simulink model "model"  (R2019a)
settings: Solver=FixedStepDiscrete  StartTime=0.0  StopTime=8  FixedStep=1/30  RelTol=1e-3  EnableMultiTasking=on
values from neighbouring files (symbols this model uses):
  A0 = 914.02    [parameter.mat]
  A1 = 12.9    [parameter.mat]
  A2 = 2028.24    [parameter.mat]
  b = 1.14    [parameter.mat]
  bpitch = 4000    [parameter.mat]
  broll = 4000    [parameter.mat]
  c = 1.14    [parameter.mat]
  C1 = 1    [parameter.mat]
  C2 = 0.34    [parameter.mat]
  C3 = 0.57    [parameter.mat]
  C4 = 0.32    [parameter.mat]
  CF = 18.7    [parameter.mat]
  f = 1.215    [parameter.mat]
  Fzt = 810    [parameter.mat]
  hs = 0.55    [parameter.mat]
  ip = 50    [parameter.mat]
  ir = 425    [parameter.mat]
  iw = 1.1    [parameter.mat]
  iz = 3136    [parameter.mat]
  Ka = 0.05    [parameter.mat]
  kpitch = 170000    [parameter.mat]
  kroll = 90000    [parameter.mat]
  m = 750    [parameter.mat]
  miudot = 0.85    [parameter.mat]
  ms = 650    [parameter.mat]
  r = 1.205    [parameter.mat]
  rw = 0.237    [parameter.mat]
  Tp = 24    [parameter.mat]
  Tw = 6    [parameter.mat]
  w = 2.28    [parameter.mat]
undefined symbols (not defined in the file or in its folder): DiscIntNeverNeededParam, Rec, SDTV, sigbuilder_block
libraries: dspmtrx3 x3, visionconversions x2, visiontextngfix x2, visiontransforms x2, fuzblock x1, dspvision x1, visionfilter x1, visionsinks x1, visionstatistics x1
(part 1 of 3)
settings Model: Creator=embb8  LastModifiedBy=embb8
settings SolverCC: PositivePriorityOrder=on
settings DataIOCC: ReturnWorkspaceOutputs=off
settings OptimizationCC: DefaultParameterBehavior=Inlined  LifeSpan=Inf  MaxStackSize=64
settings DebuggingCC: PregeneratedLibrarySubsystemCodeDiagnostic=none  SFUnexpectedBacktrackingDiag=warning  SFNoUnconditionalDefaultTransitionDiag=warning  SFExecutionAtInitializationDiag=none  ArithmeticOperatorsInVariantConditions=warning
settings HardwareCC: UseEmbeddedCoderFeatures=off  UseSimulinkCoderFeatures=off
settings SFSimCC: SimUseLocalCustomCode=off  MATLABDynamicMemAlloc=off
settings RTWCC: SystemTargetFile=ert.tlc  TemplateMakefile=ert_default_tmf  GenerateReport=on  RTWUseLocalCustomCode=off  Toolchain=GNU GCC Raspberry Pi  IncludeHyperlinkInReport=on  LaunchReport=on  GenerateTraceInfo=on  GenerateTraceReport=on  GenerateTraceReportSl=on  GenerateTraceReportSf=on  GenerateTraceReportEml=on
settings CodeAppCC: ForceParamTrailComments=on  IgnoreCustomStorageClasses=off  OperatorAnnotations=on  SimulinkDataObjDesc=on  SFDataObjDesc=on  MATLABFcnDesc=on  InsertBlockDesc=on  StateflowObjectComments=on  MATLABSourceComments=on
settings ERTTargetCC: MultiwordLength=2048  SupportNonInlinedSFcns=on  SupportVariableSizeSignals=on  InlinedParameterPlacement=NonHierarchical  ERTCustomFileTemplate=example_file_process.tlc
settings ConfigComp: CovMetricSettings=dw  CovHtmlReporting=on  CovSaveCumulativeToWorkspaceVar=on  CovSaveSingleToWorkspaceVar=on  CovExternalEMLEnable=off

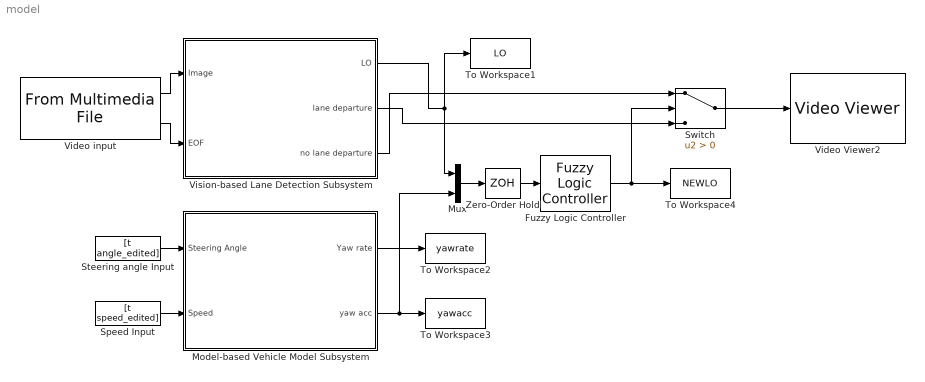
== system model ==
  Fuzzy Logic Controller : fuzblock/Fuzzy Logic  Controller  FIS=ld  OutputSampleNumber=101  DataType=double  FuzzifiedInputs=off  RuleFiringStrengths=off  RuleOutputs=off  AggregatedOutputs=off  SimulateUsing=Interpreted execution  OutOfRangeInputValueMessage=warning  NoRuleFiredMessage=warning  EmptyOutputFuzzySetMessage=warning
  Model-based Vehicle Model Subsystem : Subsystem
  Mux : Mux  Inputs=2
  Speed Input : FromWorkspace  VariableName=[t speed_edited]  SampleTime=0
  Steering angle Input : FromWorkspace  VariableName=[t angle_edited]  SampleTime=0
  Switch : Switch  Criteria=u2 > Threshold
  To Workspace1 : ToWorkspace  VariableName=LO  SampleTime=-1
      settings: Save2DSignal=2-D array (concatenate along first dimension)
  To Workspace2 : ToWorkspace  VariableName=yawrate  SampleTime=-1
      settings: Save2DSignal=2-D array (concatenate along first dimension)
  To Workspace3 : ToWorkspace  VariableName=yawacc  SampleTime=-1
      settings: Save2DSignal=2-D array (concatenate along first dimension)
  To Workspace4 : ToWorkspace  VariableName=NEWLO  SampleTime=-1
      settings: Save2DSignal=2-D array (concatenate along first dimension)
  Video Viewer2 : VideoViewer  FigPos=[617 762 372 213.6]
  Video input : dspvision/From Multimedia File  inputFilename=C:\Users\embb8\Desktop\clip20.avi  readRange=[1 Inf]  loop=on  numPlays=inf  outputStreams=Video only  videoDataType=single  audioDataType=int16  inheritSampleTime=off  userDefinedSampleTime=1/30  noAudioOutput=off  isIntensityVideo=off  fourcc=RGB  colorVideoFormat=One multidimensional signal  outputEOF=on  dataOrg=Column-major  audioFrameSize=1024  computeAudioFrameSize=off  outSamplingMode=Sample based
      settings: SourceProductName=Computer Vision Toolbox  SourceProductBaseCode=VP
  Vision-based Lane Detection Subsystem : Subsystem
  Zero-Order Hold : ZeroOrderHold  SampleTime=1/30
  wires:
  Video input/1 -> Vision-based Lane Detection Subsystem/1(Image)
  Video input/2 -> Vision-based Lane Detection Subsystem/2(EOF)
  Speed Input/1 -> Model-based Vehicle Model Subsystem/2(Speed)
  Steering angle Input/1 -> Model-based Vehicle Model Subsystem/1(Steering Angle)
  Model-based Vehicle Model Subsystem/1(Yaw rate) -> To Workspace2/1
  Vision-based Lane Detection Subsystem/1(LO) -> Mux/1, To Workspace1/1
  Vision-based Lane Detection Subsystem/2(lane departure) -> Switch/3
  Vision-based Lane Detection Subsystem/3(no lane departure) -> Switch/1
  Switch/1 -> Video Viewer2/1
  Model-based Vehicle Model Subsystem/2(yaw acc) -> Mux/2, To Workspace3/1
  Mux/1 -> Zero-Order Hold/1
  Fuzzy Logic Controller/1 -> To Workspace4/1, Switch/2
  Zero-Order Hold/1 -> Fuzzy Logic Controller/1

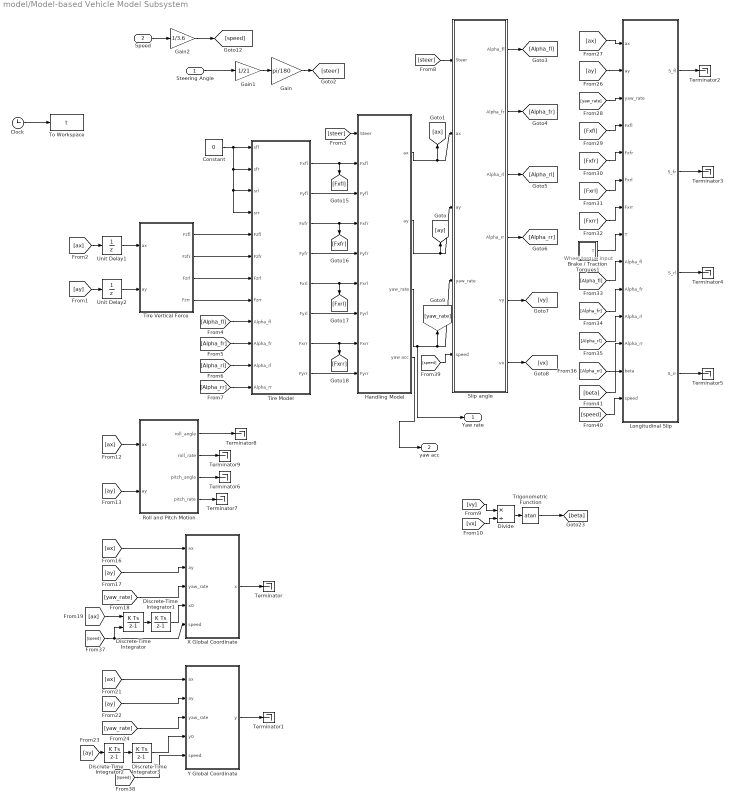
== system model/Model-based Vehicle Model Subsystem ==
  note: Wheel torque input
  Steering Angle : Inport
  Speed : Inport  Port=2
  Brake / Traction Torques1 : Subsystem
  Clock : Clock
  Constant : Constant  Value=0
  Discrete-Time Integrator : DiscreteIntegrator  InitialConditionSource=external  InitialCondition=22.222  SampleTime=-1  LimitOutput=on  LowerSaturationLimit=0  ICPrevOutput=DiscIntNeverNeededParam  ICPrevScaledInput=DiscIntNeverNeededParam
  Discrete-Time Integrator1 : DiscreteIntegrator  SampleTime=-1  LimitOutput=on  LowerSaturationLimit=0  ICPrevOutput=DiscIntNeverNeededParam  ICPrevScaledInput=DiscIntNeverNeededParam
  Discrete-Time Integrator2 : DiscreteIntegrator  SampleTime=-1  ICPrevOutput=DiscIntNeverNeededParam  ICPrevScaledInput=DiscIntNeverNeededParam
  Discrete-Time Integrator3 : DiscreteIntegrator  SampleTime=-1  ICPrevOutput=DiscIntNeverNeededParam  ICPrevScaledInput=DiscIntNeverNeededParam
  Divide : Product  Inputs=*/
  Gain : Gain  Gain=pi/180
  Gain1 : Gain  Gain=1/21
  Gain2 : Gain  Gain=1/3.6
  "Handling Model " : Subsystem
  Longitudinal Slip : Subsystem
  Roll and Pitch Motion : Subsystem
  "Slip angle " : Subsystem
  Terminator{,1..9} (10 alike) : Terminator
  Tire Model : Subsystem
  Tire Vertical Force : Subsystem
  To Workspace : ToWorkspace  VariableName=t  SampleTime=-1
  Trigonometric Function : Trigonometry  Operator=atan
  Unit Delay1 : UnitDelay  SampleTime=1/30  HasFrameUpgradeWarning=on
  Unit Delay2 : UnitDelay  SampleTime=1/30  HasFrameUpgradeWarning=on
  X Global Coordinate : Subsystem
  Y Global Coordinate : Subsystem
  Yaw rate : Outport
  yaw acc : Outport  Port=2
  wires:
  [speed] -> X Global Coordinate/5(speed), Discrete-Time Integrator/2
  [speed] -> Longitudinal Slip/14(speed)
  [Fxrr] -> Longitudinal Slip/7(Fxrr)
  Gain1/1 -> Gain/1
  "Slip angle "/3(Alpha_rl) -> [Alpha_rl]
  Longitudinal Slip/4(S_rr) -> Terminator5/1
  [ax] -> Longitudinal Slip/1(ax)
  Discrete-Time Integrator3/1 -> Y Global Coordinate/4(y0)
  [speed] -> Y Global Coordinate/5(speed)
  [ay] -> X Global Coordinate/2(ay)
  Longitudinal Slip/3(S_rl) -> Terminator4/1
  [Fxfl] -> Longitudinal Slip/4(Fxfl)
  Tire Model/6(Fyrl) -> "Handling Model "/7(Fyrl)
  Y Global Coordinate/1(y) -> Terminator1/1
  [Alpha_rr] -> Longitudinal Slip/12(Alpha_rr)
  Unit Delay2/1 -> Tire Vertical Force/2(ay)
  Tire Vertical Force/2(Fzfr) -> Tire Model/6(Fzfr)
  [Alpha_rr] -> Tire Model/12(Alpha_rr)
  Clock/1 -> To Workspace/1
  Brake / Traction Torques1/1(T) -> Longitudinal Slip/8(T)
  [ax] -> Roll and Pitch Motion/1(ax)
  [ax] -> X Global Coordinate/1(ax)
  Constant/1 -> Tire Model/1(sfl), Tire Model/2(sfr), Tire Model/3(srl), Tire Model/4(srr)
  Roll and Pitch Motion/1(roll_angle) -> Terminator8/1
  [Fxrl] -> Longitudinal Slip/6(Fxrl)
  [ay] -> Longitudinal Slip/2(ay)
  Tire Vertical Force/1(Fzfl) -> Tire Model/5(Fzfl)
  Roll and Pitch Motion/4(pitch_rate) -> Terminator7/1
  [Fxfr] -> Longitudinal Slip/5(Fxfr)
  [yaw_rate] -> Y Global Coordinate/3(yaw_rate)
  [Alpha_fr] -> Longitudinal Slip/10(Alpha_fr)
  Roll and Pitch Motion/3(pitch_angle) -> Terminator6/1
  [Alpha_fl] -> Longitudinal Slip/9(Alpha_fl)
  [Alpha_fl] -> Tire Model/9(Alpha_fl)
  [Alpha_rl] -> Longitudinal Slip/11(Alpha_rl)
  [yaw_rate] -> Longitudinal Slip/3(yaw_rate)
  [yaw_rate] -> X Global Coordinate/3(yaw_rate)
  [beta] -> Longitudinal Slip/13(beta)
  X Global Coordinate/1(x) -> Terminator/1
  [speed] -> "Slip angle "/5(speed)
  [ax] -> Y Global Coordinate/1(ax)
  "Slip angle "/6(vx) -> [vx]
  "Slip angle "/4(Alpha_rr) -> [Alpha_rr]
  [ay] -> Discrete-Time Integrator2/1
  Longitudinal Slip/2(S_fr) -> Terminator3/1
  "Handling Model "/1(ax) -> [ax], "Slip angle "/2(ax)
  Discrete-Time Integrator/1 -> Discrete-Time Integrator1/1
  [steer] -> "Handling Model "/1(Steer)
  "Slip angle "/2(Alpha_fr) -> [Alpha_fr]
  [Alpha_fr] -> Tire Model/10(Alpha_fr)
  [ax] -> Unit Delay1/1
  [ax] -> Discrete-Time Integrator/1
  [ay] -> Roll and Pitch Motion/2(ay)
  Roll and Pitch Motion/2(roll_rate) -> Terminator9/1
  Tire Model/1(Fxfl) -> "Handling Model "/2(Fxfl), [Fxfl]
  Discrete-Time Integrator2/1 -> Discrete-Time Integrator3/1
  Tire Model/8(Fyrr) -> "Handling Model "/9(Fyrr)
  "Handling Model "/2(ay) -> [ay], "Slip angle "/3(ay)
  Gain/1 -> [steer]
  [ay] -> Unit Delay2/1
  [Alpha_rl] -> Tire Model/11(Alpha_rl)
  [ay] -> Y Global Coordinate/2(ay)
  "Slip angle "/1(Alpha_fl) -> [Alpha_fl]
  "Slip angle "/5(vy) -> [vy]
  Tire Model/7(Fxrr) -> "Handling Model "/8(Fxrr), [Fxrr]
  [steer] -> "Slip angle "/1(Steer)
  Tire Vertical Force/4(Fzrr) -> Tire Model/8(Fzrr)
  Longitudinal Slip/1(S_fl) -> Terminator2/1
  Tire Model/2(Fyfl) -> "Handling Model "/3(Fyfl)
  Tire Model/4(Fyfr) -> "Handling Model "/5(Fyfr)
  Discrete-Time Integrator1/1 -> X Global Coordinate/4(x0)
  Tire Model/3(Fxfr) -> "Handling Model "/4(Fxfr), [Fxfr]
  Tire Vertical Force/3(Fzrl) -> Tire Model/7(Fzrl)
  Unit Delay1/1 -> Tire Vertical Force/1(ax)
  Tire Model/5(Fxrl) -> "Handling Model "/6(Fxrl), [Fxrl]
  Speed/1 -> Gain2/1
  Steering Angle/1 -> Gain1/1
  "Handling Model "/3(yaw_rate) -> Yaw rate/1, "Slip angle "/4(yaw_rate), [yaw_rate]
  [vy] -> Divide/1
  [vx] -> Divide/2
  Divide/1 -> Trigonometric Function/1
  Trigonometric Function/1 -> [beta]
  Gain2/1 -> [speed]
  "Handling Model "/4(yaw acc) -> yaw acc/1

== system model/Vision-based Lane Detection Subsystem ==
  note: |
      | |
      | |
      | |
      | |
      | |
      | y(180)
  note: _____________>x(320)
  note: x11 y12 x12 y12
      | x21 y21 x22 y22
  note: Plan to do list:
      | 1. Vision lateral offset (Done)
      | 2. Benchmark with other edge-based lane detection algorithm.
      | 3. Vehicle Model (Driver Model) lateral offset
      | 4. Steering Angle and Speed Sensor integrate into vehicle model.
      | 5. Integrate vision model and vehicle model with fuzzy system to compare respective lateral offset for lane warning.
  Image : Inport
  EOF : Inport  Port=2
  2-D FIR Filter : visionfilter/2-D FIR Filter  separable=off  filtSrc=Specify via dialog  filterMtrx=[-1 0 1]  verticalFilter=[4 0]  horizontalFilter=[4 0]  outSize=Full  padType=Replicate  padSrc=Specify via dialog  padVal=0  method=Convolution  firstCoeffMode=Specify word length  firstCoeffWordLength=16  firstCoeffFracLength=14  firstCoeffSignedness=Signed  firstCoeffLastDataTypeStr=fixdt(1,16)  outputSignedness=Auto  accumLastDataTypeStr=Inherit: Same as product output  prodOutputMode=Binary point scaling  prodOutputWordLength=32  prodOutputFracLength=10  prodOutputLastDataTypeStr=fixdt([],32,10)  roundingMode=Floor  overflowMode=on  firstCoeffDataTypeStr=fixdt(1,16)  firstCoeffMin=[]  firstCoeffMax=[]  prodOutputDataTypeStr=fixdt([],32,10)  accumDataTypeStr=Inherit: Same as product output  outputMin=[]  outputMax=[]
      settings: SourceProductName=Computer Vision Toolbox  SourceProductBaseCode=VP
  After : Display
  Clip image : dspmtrx3/Submatrix  RowSpan=Range of rows  RowStartMode=Index  RowStartIndex=u+1  RowEndMode=Last  RowEndIndex=1  ColSpan=All columns  ColStartMode=First  ColStartIndex=1  ColEndMode=Last  ColEndIndex=1
  Color Space Conversion : visionconversions/Color Space  Conversion  conversion=Obsolete  conversionActive=R'G'B' to intensity  wp_str=D65  rec=Rec. 601 (SDTV)  sys=1125/60/2:1  imagePorts=One multidimensional signal
  Draw Shapes : visiontextngfix/Draw Shapes  shape=Lines  fill=on  lineWidth=3  fillClrSource=Specify via dialog  display=User-specified value  intensity=200  color=[255 0 0]  opacity=0.6  viewport=Entire image  antialiasing=on  inType=Obsolete  imagePorts=One multidimensional signal  roundingMode=Floor  overflowMode=off  memoryMode=Specify word length  memoryWordLength=16  prodOutputMode=Binary point scaling  prodOutputWordLength=32  prodOutputFracLength=14  prodOutputSlope=2^-14  accumSlope=2^-14  memoryFracLength=14
      settings: SourceProductName=Computer Vision Toolbox
  Frame Rate Display : visionsinks/Frame Rate Display  UpdateRate=1
      settings: SourceProductName=Computer Vision Toolbox  SourceProductBaseCode=VP
  Hough Transform : Subsystem
  Image thresholding : visionconversions/Autothreshold  operator=>  threshOut=off  effMetricOut=off  userDefinedRange=off  umin=0  umax=255  outOfRngOpt=Warn and saturate  scaleThreshold=off  scaleFactor=1  roundingMode=Floor  overflowMode=off  P1Mode=Specify word length  P1WordLength=32  P1FracLength=30  P1Slope=2^-30  A1Slope=2^-30  P2Mode=Specify word length  P2WordLength=32  P2FracLength=22  P2Slope=2^-22  A2Slope=2^-22  P3Mode=Specify word length  P3WordLength=32  P3FracLength=14  P3Slope=2^-14  A3Slope=2^-14  P4Mode=Binary point scaling  P4WordLength=32  P4FracLength=15  P4Slope=2^-15  A4Slope=2^-4  Q1Mode=Specify word length  Q1WordLength=32  Q1FracLength=16  Q1Slope=2^-16  EMMode=Specify word length  EMWordLength=16  EMFracLength=14  EMSlope=2^-14
      settings: SourceProductName=Computer Vision Toolbox  SourceProductBaseCode=VP
  Insert Text : visiontextngfix/Insert Text  inputType=Obsolete  theText='Lane Departure'  getTextLocFrom=Specify via dialog  textLoc=[120 60]  getTextColorFrom=Specify via dialog  textColor=[255 0 0]  getTextIntensityFrom=Specify via dialog  textIntensity=0  getTextOpacityFrom=Specify via dialog  textOpacity=1.0  dummyVar2=0  dummyVar3=0  dummyVar4=0  imagePorts=One multidimensional signal  isInputTransposed=off  fontFace=LucidaSansRegular  dummyVar1=0  blockFontSize=20  antiAliased=on
      settings: SourceProductName=Computer Vision Toolbox  SourceProductBaseCode=VP
  Saturation : Saturate  UpperLimit=1  LowerLimit=0
  Selector3 : Selector  NumberOfDimensions=2  InputPortWidth=3  IndexOptions=Select all,Index vector (dialog)  Indices=[2 1],[2 1 4 3]  OutputSizes=1,1
  Selector4 : Selector  NumberOfDimensions=2  InputPortWidth=3  IndexOptions=Index vector (dialog),Select all  Indices=[2 1 4 3],1  OutputSizes=1,1
  Stop Simulation : Stop
  Subsystem : Subsystem
  Transpose : Math  Operator=transpose  SaturateOnIntegerOverflow=on
  Transpose1 : Math  Operator=transpose  SaturateOnIntegerOverflow=on
  coordinate mapping : Subsystem
  lateral offset : Subsystem
  offset (+88) : Subsystem
  LO : Outport
  lane departure : Outport  Port=2
  no lane departure : Outport  Port=3
  wires:
  Subsystem/1(Out1) -> coordinate mapping/1(In1), After/1
  EOF/1 -> Stop Simulation/1
  2-D FIR Filter/1 -> Saturation/1
  Saturation/1 -> Image thresholding/1
  Transpose1/1 -> Subsystem/1(In1), Draw Shapes/2
  Image thresholding/1 -> Hough Transform/1(In1)
  offset (+88)/2(left) -> lateral offset/2(left)
  Hough Transform/1(Out1) -> Selector3/1
  Image/1 -> Draw Shapes/1, Color Space Conversion/1
  offset (+88)/3(right) -> lateral offset/1(right)
  Transpose/1 -> offset (+88)/1(In1)
  offset (+88)/1(Out1) -> Selector4/1
  Clip image/1 -> Hough Transform/2(ref_I), 2-D FIR Filter/1
  Selector4/1 -> Transpose1/1
  Draw Shapes/1 -> no lane departure/1, Insert Text/1, Frame Rate Display/1
  Selector3/1 -> Transpose/1
  Color Space Conversion/1 -> Clip image/1
  Insert Text/1 -> lane departure/1
  lateral offset/1(lateral offset) -> LO/1

== system model/Model-based Vehicle Model Subsystem/Brake // Traction Torques1 ==
  note: T negative for braking
      | T positive for traction
  BRAKE : Subsystem  Tag=STV Subsys  LoadFcn=sigbuilder_block('load');  StartFcn=sigbuilder_block('start');  StopFcn=sigbuilder_block('stop');  ClipboardFcn=sigbuilder_block('clipboard');  mask(Sigbuilder block){tuvar=[0:10]}
      mask help: Sigbuilder GUI
      mask init:
      | if ~strcmp(get_param(bdroot(gcbh),'SimulationStatus'),'stopped') tuvar = sigbuilder_block('maskInit'); end
      settings: CopyFcn=sigbuilder_block('copy');  DeleteFcn=sigbuilder_block('delete');  ModelCloseFcn=sigbuilder_block('modelClose');  PreSaveFcn=sigbuilder_block('preSave');  PauseFcn=sigbuilder_block('pause')  ContinueFcn=sigbuilder_block('continue')  NameChangeFcn=sigbuilder_block('namechange');  OpenFcn=sigbuilder_block('open',[51.75 84.75 550.5 363.75 ]);  CloseFcn=sigbuilder_block('close');
      mask Display: plot(0, 0, 100, 100,[2, 2, 32, 32, 2], [68, 8, 8, 68, 68],[32, 2], [38, 38], [32, 19, 2],[53, 60, 44], [32, 17, 17, 2],[16, 16, 31, 31]);txt = getActiveGroup(gcbh);text(2, 100, txt,'verticalAlignment', 'top');
  Bus Creator : BusCreator  Inputs=4
  Gain : Gain  Gain=300
  Gain1 : Gain  Gain=300
  Gain{8..11} (4 alike) : Gain  Gain=-6
  Gain12 : Gain  Gain=0
  Gain2 : Gain  Gain=0
  Gain3 : Gain  Gain=0
  Gain4 : Gain  Gain=200
  Gain5 : Gain  Gain=200
  Gain6 : Gain  Gain=80
  Gain7 : Gain  Gain=80
  Scope : Scope
  Switch : Switch  Criteria=u2 > Threshold  Threshold=199
  Switch1 : Switch  Criteria=u2 > Threshold  Threshold=199
  Switch2 : Switch  Criteria=u2 > Threshold  Threshold=-1
  Switch3 : Switch  Criteria=u2 > Threshold  Threshold=-1
  THROTTLE1 : Subsystem  Tag=STV Subsys  LoadFcn=sigbuilder_block('load');  StartFcn=sigbuilder_block('start');  StopFcn=sigbuilder_block('stop');  ClipboardFcn=sigbuilder_block('clipboard');  mask(Sigbuilder block){tuvar=[0:10]}
      mask help: Sigbuilder GUI
      mask init:
      | if ~strcmp(get_param(bdroot(gcbh),'SimulationStatus'),'stopped') tuvar = sigbuilder_block('maskInit'); end
      settings: CopyFcn=sigbuilder_block('copy');  DeleteFcn=sigbuilder_block('delete');  ModelCloseFcn=sigbuilder_block('modelClose');  PreSaveFcn=sigbuilder_block('preSave');  PauseFcn=sigbuilder_block('pause')  ContinueFcn=sigbuilder_block('continue')  NameChangeFcn=sigbuilder_block('namechange');  OpenFcn=sigbuilder_block('open',[252 113.25 550.5 363.75 ]);  CloseFcn=sigbuilder_block('close');
      mask Display: plot(0, 0, 100, 100,[2, 2, 32, 32, 2], [68, 8, 8, 68, 68],[32, 2], [38, 38], [32, 19, 2],[53, 60, 44], [32, 17, 17, 2],[16, 16, 31, 31]);txt = getActiveGroup(gcbh);text(2, 100, txt,'verticalAlignment', 'top');
  T : Outport
  wires:
  Gain11/1 -> Gain7/1, Switch3/2
  Gain9/1 -> Gain6/1, Switch2/2
  Gain10/1 -> Gain5/1
  Bus Creator/1 -> T/1, Scope/1
  Gain8/1 -> Gain4/1
  BRAKE/1(Signal 1) -> Gain11/1, Gain9/1, Gain10/1, Gain8/1
  THROTTLE1/1(Signal 1) -> Gain12/1
  Switch/1 -> Bus Creator/1
  Switch1/1 -> Bus Creator/2
  Switch2/1 -> Bus Creator/3
  Gain/1 -> Switch/1, Switch/2
  Gain4/1 -> Switch/3
  Gain1/1 -> Switch1/1, Switch1/2
  Gain5/1 -> Switch1/3
  Gain2/1 -> Switch2/1
  Gain6/1 -> Switch2/3
  Gain3/1 -> Switch3/1
  Gain7/1 -> Switch3/3
  Switch3/1 -> Bus Creator/4
  Gain12/1 -> Gain/1, Gain1/1, Gain2/1, Gain3/1

== system model/Model-based Vehicle Model Subsystem/Handling Model  ==
  Steer : Inport
  Fxfl : Inport  Port=2
  Fyfl : Inport  Port=3
  Fxfr : Inport  Port=4
  Fyfr : Inport  Port=5
  Fxrl : Inport  Port=6
  Fyrl : Inport  Port=7
  Fxrr : Inport  Port=8
  Fyrr : Inport  Port=9
  "Lateral " : Subsystem
  "Longitudinal " : Subsystem
  "Yaw  " : Subsystem
  ax : Outport
  ay : Outport  Port=2
  yaw_rate : Outport  Port=3
  yaw acc : Outport  Port=4
  wires:
  Steer/1 -> "Longitudinal "/1(Steer), "Yaw  "/1(Steer), "Lateral "/1(Steer)
  Fxfl/1 -> "Longitudinal "/2(Fxfl), "Yaw  "/2(Fxfl), "Lateral "/2(Fxfl)
  Fyfl/1 -> "Longitudinal "/3(Fyfl), "Yaw  "/3(Fyfl), "Lateral "/3(Fyfl)
  Fxfr/1 -> "Longitudinal "/4(Fxfr), "Yaw  "/4(Fxfr), "Lateral "/4(Fxfr)
  Fyfr/1 -> "Longitudinal "/5(Fyfr), "Yaw  "/5(Fyfr), "Lateral "/5(Fyfr)
  Fxrl/1 -> "Yaw  "/6(Fxrl), "Longitudinal "/6(Fxrl)
  Fyrl/1 -> "Yaw  "/7(Fyrl), "Lateral "/6(Fyrl)
  "Longitudinal "/1(ax) -> ax/1
  "Lateral "/1(ay) -> ay/1
  "Yaw  "/1(yaw_rate) -> yaw_rate/1
  Fxrr/1 -> "Yaw  "/8(Fxrr), "Longitudinal "/7(Fxrr)
  Fyrr/1 -> "Yaw  "/9(Fyrr), "Lateral "/7(Fyrr)
  "Yaw  "/2(yaw acc) -> yaw acc/1

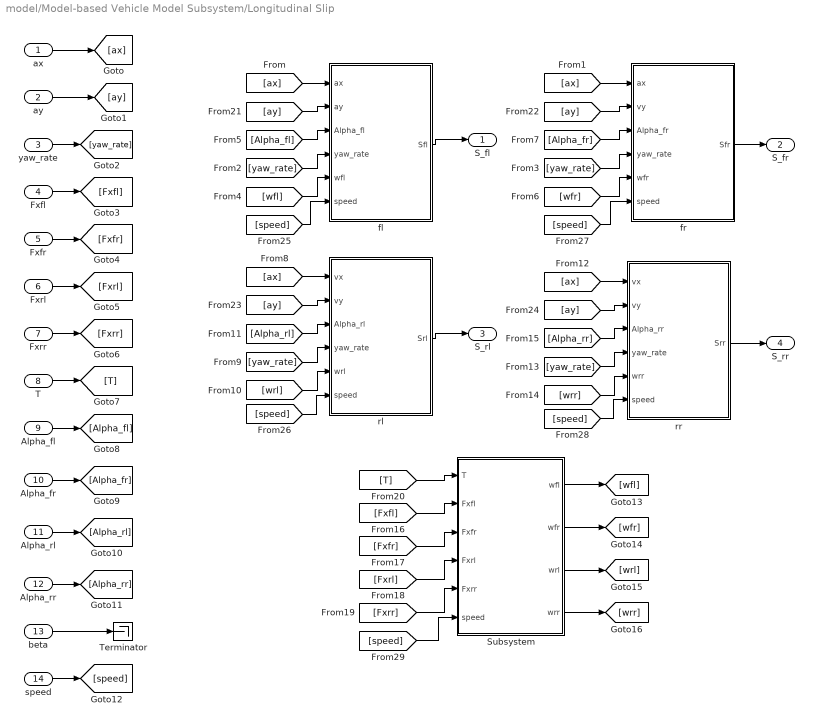
== system model/Model-based Vehicle Model Subsystem/Longitudinal Slip ==
  ax : Inport
  ay : Inport  Port=2
  yaw_rate : Inport  Port=3
  Fxfl : Inport  Port=4
  Fxfr : Inport  Port=5
  Fxrl : Inport  Port=6
  Fxrr : Inport  Port=7
  T : Inport  Port=8
  Alpha_fl : Inport  Port=9
  Alpha_fr : Inport  Port=10
  Alpha_rl : Inport  Port=11
  Alpha_rr : Inport  Port=12
  beta : Inport  Port=13
  speed : Inport  Port=14
  Subsystem : Subsystem
  Terminator : Terminator
  fl : Subsystem
  fr : Subsystem
  rl : Subsystem
  rr : Subsystem
  S_fl : Outport
  S_fr : Outport  Port=2
  S_rl : Outport  Port=3
  S_rr : Outport  Port=4
  wires:
  ax/1 -> [ax]
  ay/1 -> [ay]
  yaw_rate/1 -> [yaw_rate]
  Fxfl/1 -> [Fxfl]
  Fxfr/1 -> [Fxfr]
  Fxrl/1 -> [Fxrl]
  Fxrr/1 -> [Fxrr]
  T/1 -> [T]
  Alpha_fl/1 -> [Alpha_fl]
  Alpha_fr/1 -> [Alpha_fr]
  Alpha_rl/1 -> [Alpha_rl]
  Alpha_rr/1 -> [Alpha_rr]
  fl/1(Sfl) -> S_fl/1
  [ax] -> fl/1(ax)
  [yaw_rate] -> fl/4(yaw_rate)
  [wfl] -> fl/5(wfl)
  beta/1 -> Terminator/1
  [Alpha_fl] -> fl/3(Alpha_fl)
  fr/1(Sfr) -> S_fr/1
  [wfr] -> fr/5(wfr)
  rl/1(Srl) -> S_rl/1
  [wrl] -> rl/5(wrl)
  rr/1(Srr) -> S_rr/1
  [wrr] -> rr/5(wrr)
  [Fxfl] -> Subsystem/2(Fxfl)
  [Fxfr] -> Subsystem/3(Fxfr)
  [Fxrl] -> Subsystem/4(Fxrl)
  [Fxrr] -> Subsystem/5(Fxrr)
  [T] -> Subsystem/1(T)
  Subsystem/1(wfl) -> [wfl]
  Subsystem/2(wfr) -> [wfr]
  Subsystem/3(wrl) -> [wrl]
  Subsystem/4(wrr) -> [wrr]
  [ay] -> fl/2(ay)
  [ax] -> fr/1(ax)
  [ay] -> fr/2(vy)
  [Alpha_fr] -> fr/3(Alpha_fr)
  [yaw_rate] -> fr/4(yaw_rate)
  [ax] -> rl/1(vx)
  [ay] -> rl/2(vy)
  [Alpha_rl] -> rl/3(Alpha_rl)
  [yaw_rate] -> rl/4(yaw_rate)
  [ax] -> rr/1(vx)
  [ay] -> rr/2(vy)
  [Alpha_rr] -> rr/3(Alpha_rr)
  [yaw_rate] -> rr/4(yaw_rate)
  speed/1 -> [speed]
  [speed] -> fl/6(speed)
  [speed] -> rl/6(speed)
  [speed] -> fr/6(speed)
  [speed] -> rr/6(speed)
  [speed] -> Subsystem/6(speed)

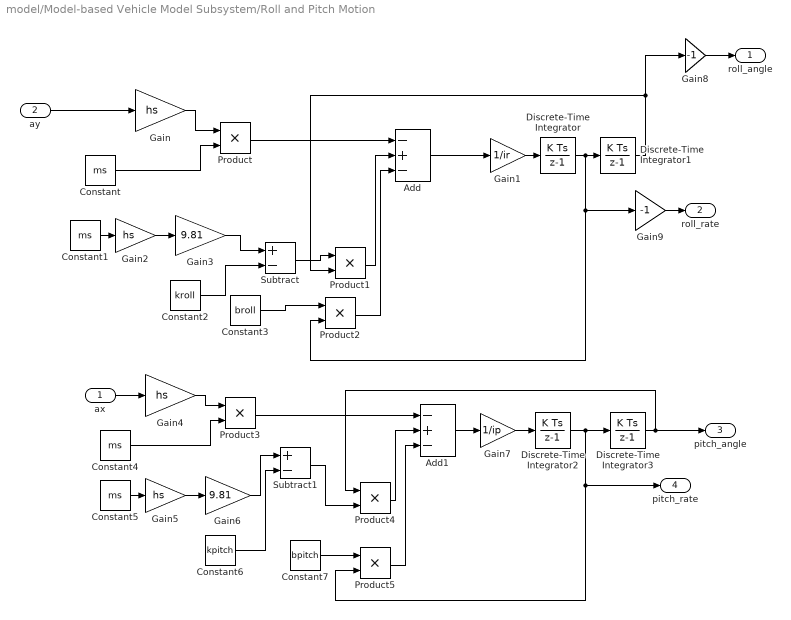
== system model/Model-based Vehicle Model Subsystem/Roll and Pitch Motion ==
  ax : Inport
  ay : Inport  Port=2
  Add : Sum  Inputs=-+-
  Add1 : Sum  Inputs=-+-
  Constant{,1,4..5} (4 alike) : Constant  Value=ms
  Constant2 : Constant  Value=kroll
  Constant3 : Constant  Value=broll
  Constant6 : Constant  Value=kpitch
  Constant7 : Constant  Value=bpitch
  Discrete-Time Integrator{,1..3} (4 alike) : DiscreteIntegrator  SampleTime=-1  ICPrevOutput=DiscIntNeverNeededParam  ICPrevScaledInput=DiscIntNeverNeededParam
  Gain{,2,4..5} (4 alike) : Gain  Gain=hs
  Gain1 : Gain  Gain=1/ir
  Gain3 : Gain  Gain=9.81
  Gain6 : Gain  Gain=9.81
  Gain7 : Gain  Gain=1/ip
  Gain8 : Gain  Gain=-1
  Gain9 : Gain  Gain=-1
  Product{,1..5} (6 alike) : Product  RndMeth=Zero
  Subtract : Sum  Inputs=+-
  Subtract1 : Sum  Inputs=+-
  roll_angle : Outport
  roll_rate : Outport  Port=2
  pitch_angle : Outport  Port=3
  pitch_rate : Outport  Port=4
  wires:
  ay/1 -> Gain/1
  Constant/1 -> Product/2
  Gain/1 -> Product/1
  Constant1/1 -> Gain2/1
  Gain2/1 -> Gain3/1
  Gain3/1 -> Subtract/1
  Constant2/1 -> Subtract/2
  Product/1 -> Add/1
  Subtract/1 -> Product1/1
  Add/1 -> Gain1/1
  Gain1/1 -> Discrete-Time Integrator/1
  Discrete-Time Integrator/1 -> Product2/2, Gain9/1, Discrete-Time Integrator1/1
  Discrete-Time Integrator1/1 -> Product1/2, Gain8/1
  Product1/1 -> Add/2
  Constant3/1 -> Product2/1
  Product2/1 -> Add/3
  ax/1 -> Gain4/1
  Gain4/1 -> Product3/1
  Constant4/1 -> Product3/2
  Product3/1 -> Add1/1
  Constant5/1 -> Gain5/1
  Gain5/1 -> Gain6/1
  Gain6/1 -> Subtract1/1
  Constant6/1 -> Subtract1/2
  Product4/1 -> Add1/2
  Add1/1 -> Gain7/1
  Gain7/1 -> Discrete-Time Integrator2/1
  Discrete-Time Integrator2/1 -> Discrete-Time Integrator3/1, Product5/2, pitch_rate/1
  Discrete-Time Integrator3/1 -> Product4/1, pitch_angle/1
  Constant7/1 -> Product5/1
  Product5/1 -> Add1/3
  Subtract1/1 -> Product4/2
  Gain8/1 -> roll_angle/1
  Gain9/1 -> roll_rate/1

== system model/Model-based Vehicle Model Subsystem/Slip angle  ==
  Steer : Inport
  ax : Inport  Port=2
  ay : Inport  Port=3
  yaw_rate : Inport  Port=4
  speed : Inport  Port=5
  Subsystem1 : Subsystem
  yaw effect motion : Subsystem
  Alpha_fl : Outport
  Alpha_fr : Outport  Port=2
  Alpha_rl : Outport  Port=3
  Alpha_rr : Outport  Port=4
  vy : Outport  Port=5
  vx : Outport  Port=6
  wires:
  ax/1 -> yaw effect motion/1(ax)
  ay/1 -> yaw effect motion/2(ay)
  yaw_rate/1 -> Subsystem1/4(yaw_rate), yaw effect motion/3(yaw_rate)
  yaw effect motion/1(vx) -> Subsystem1/2(vx), vx/1
  yaw effect motion/2(vy) -> Subsystem1/3(vy), vy/1
  Steer/1 -> Subsystem1/1(Steer)
  Subsystem1/1(Alpha_fl) -> Alpha_fl/1
  Subsystem1/2(Alpha_fr) -> Alpha_fr/1
  Subsystem1/3(Alpha_rl) -> Alpha_rl/1
  Subsystem1/4(Alpha_rr) -> Alpha_rr/1
  speed/1 -> yaw effect motion/4(speed)

== system model/Model-based Vehicle Model Subsystem/Tire Model ==
  sfl : Inport
  sfr : Inport  Port=2
  srl : Inport  Port=3
  srr : Inport  Port=4
  Fzfl : Inport  Port=5
  Fzfr : Inport  Port=6
  Fzrl : Inport  Port=7
  Fzrr : Inport  Port=8
  Alpha_fl : Inport  Port=9
  Alpha_fr : Inport  Port=10
  Alpha_rl : Inport  Port=11
  Alpha_rr : Inport  Port=12
  Subsystem : Subsystem
  Subsystem1 : Subsystem
  Subsystem2 : Subsystem
  Subsystem3 : Subsystem
  Fxfl : Outport
  Fyfl : Outport  Port=2
  Fxfr : Outport  Port=3
  Fyfr : Outport  Port=4
  Fxrl : Outport  Port=5
  Fyrl : Outport  Port=6
  Fxrr : Outport  Port=7
  Fyrr : Outport  Port=8
  wires:
  sfl/1 -> Subsystem/1(sfl)
  Fzfl/1 -> Subsystem/2(Fzfl)
  Alpha_fl/1 -> Subsystem/3(Alpha_fl)
  Subsystem/1(Fxfl) -> Fxfl/1
  Subsystem/2(Fyfl) -> Fyfl/1
  Subsystem1/1(Fxfr) -> Fxfr/1
  Subsystem1/2(Fyfr) -> Fyfr/1
  sfr/1 -> Subsystem1/1(sfr)
  Fzfr/1 -> Subsystem1/2(Fzfr)
  Alpha_fr/1 -> Subsystem1/3(Alpha_fr)
  Subsystem2/1(Fxrl) -> Fxrl/1
  Subsystem2/2(Fyrl) -> Fyrl/1
  srl/1 -> Subsystem2/1(srl)
  Fzrl/1 -> Subsystem2/2(Fzrl)
  Alpha_rl/1 -> Subsystem2/3(Alpha_rl)
  Subsystem3/1(Fxrr) -> Fxrr/1
  Subsystem3/2(Fyrr) -> Fyrr/1
  srr/1 -> Subsystem3/1(srr)
  Fzrr/1 -> Subsystem3/2(Fzrr)
  Alpha_rr/1 -> Subsystem3/3(Alpha_rr)

== system model/Model-based Vehicle Model Subsystem/Tire Vertical Force ==
  ax : Inport
  ay : Inport  Port=2
  Subsystem1 : Subsystem
  Fzfl : Outport
  Fzfr : Outport  Port=2
  Fzrl : Outport  Port=3
  Fzrr : Outport  Port=4
  wires:
  ax/1 -> Subsystem1/1(ax)
  ay/1 -> Subsystem1/2(ay)
  Subsystem1/1(Fzfl) -> Fzfl/1
  Subsystem1/2(Fzfr) -> Fzfr/1
  Subsystem1/3(Fzrl) -> Fzrl/1
  Subsystem1/4(Fzrr) -> Fzrr/1

== system model/Model-based Vehicle Model Subsystem/X Global Coordinate ==
  ax : Inport
  ay : Inport  Port=2
  yaw_rate : Inport  Port=3
  x0 : Inport  Port=4
  speed : Inport  Port=5
  Add : Sum
  Discrete-Time Integrator : DiscreteIntegrator  SampleTime=-1  ICPrevOutput=DiscIntNeverNeededParam  ICPrevScaledInput=DiscIntNeverNeededParam
  Discrete-Time Integrator1 : DiscreteIntegrator  InitialConditionSource=external  InitialCondition=22.222  SampleTime=-1  LimitOutput=on  LowerSaturationLimit=0  ICPrevOutput=DiscIntNeverNeededParam  ICPrevScaledInput=DiscIntNeverNeededParam
  Discrete-Time Integrator2 : DiscreteIntegrator  SampleTime=-1  ICPrevOutput=DiscIntNeverNeededParam  ICPrevScaledInput=DiscIntNeverNeededParam
  Discrete-Time Integrator3 : DiscreteIntegrator  SampleTime=-1  ICPrevOutput=DiscIntNeverNeededParam  ICPrevScaledInput=DiscIntNeverNeededParam
  Product : Product  RndMeth=Zero
  Product1 : Product  RndMeth=Zero
  Subtract : Sum  Inputs=+-
  Trigonometric Function : Trigonometry  Operator=cos
  Trigonometric Function1 : Trigonometry
  x : Outport
  wires:
  ax/1 -> Discrete-Time Integrator1/1
  ay/1 -> Discrete-Time Integrator2/1
  Discrete-Time Integrator1/1 -> Product/1
  yaw_rate/1 -> Discrete-Time Integrator3/1
  Discrete-Time Integrator3/1 -> Trigonometric Function/1, Trigonometric Function1/1
  Trigonometric Function/1 -> Product/2
  Discrete-Time Integrator2/1 -> Product1/1
  Trigonometric Function1/1 -> Product1/2
  Product1/1 -> Subtract/2
  Product/1 -> Subtract/1
  Subtract/1 -> Discrete-Time Integrator/1
  Discrete-Time Integrator/1 -> Add/1
  x0/1 -> Add/2
  Add/1 -> x/1
  speed/1 -> Discrete-Time Integrator1/2

== system model/Model-based Vehicle Model Subsystem/Y Global Coordinate ==
  ax : Inport
  ay : Inport  Port=2
  yaw_rate : Inport  Port=3
  y0 : Inport  Port=4
  speed : Inport  Port=5
  Add : Sum
  Discrete-Time Integrator : DiscreteIntegrator  InitialConditionSource=external  InitialCondition=22.222  SampleTime=-1  LimitOutput=on  LowerSaturationLimit=0  ICPrevOutput=DiscIntNeverNeededParam  ICPrevScaledInput=DiscIntNeverNeededParam
  Discrete-Time Integrator1 : DiscreteIntegrator  SampleTime=-1  ICPrevOutput=DiscIntNeverNeededParam  ICPrevScaledInput=DiscIntNeverNeededParam
  Discrete-Time Integrator2 : DiscreteIntegrator  SampleTime=-1  ICPrevOutput=DiscIntNeverNeededParam  ICPrevScaledInput=DiscIntNeverNeededParam
  Discrete-Time Integrator3 : DiscreteIntegrator  SampleTime=-1  ICPrevOutput=DiscIntNeverNeededParam  ICPrevScaledInput=DiscIntNeverNeededParam
  Product : Product  RndMeth=Zero
  Product1 : Product  RndMeth=Zero
  Subtract : Sum
  Trigonometric Function : Trigonometry
  Trigonometric Function1 : Trigonometry  Operator=cos
  y : Outport
  wires:
  ax/1 -> Discrete-Time Integrator/1
  ay/1 -> Discrete-Time Integrator1/1
  Discrete-Time Integrator/1 -> Product/1
  yaw_rate/1 -> Discrete-Time Integrator2/1
  Discrete-Time Integrator2/1 -> Trigonometric Function/1, Trigonometric Function1/1
  Discrete-Time Integrator1/1 -> Product1/1
  Product1/1 -> Subtract/2
  Product/1 -> Subtract/1
  Subtract/1 -> Discrete-Time Integrator3/1
  Discrete-Time Integrator3/1 -> Add/1
  y0/1 -> Add/2
  Add/1 -> y/1
  Trigonometric Function/1 -> Product/2
  Trigonometric Function1/1 -> Product1/2
  speed/1 -> Discrete-Time Integrator/2

== system model/Vision-based Lane Detection Subsystem/Hough Transform ==
  note: Wipe out Hamtrix with
      | theta >=  70deg
  note: Wipe out Hamtrix with
      | theta <  -70deg
  In1 : Inport
  ref_I : Inport  Port=2
  Hough Lines : visiontransforms/Hough Lines  sineCompMethod=Trigonometric function  thetaRes=pi/180  roundingMode=Nearest  overflowMode=on  firstCoeffMode=Specify word length  firstCoeffWordLength=16  prodOutputMode=Binary point scaling  prodOutputWordLength=32  prodOutputFracLength=16  prodOutputSlope=2^-16  accumSlope=2^-16  firstCoeffFracLength=15
      settings: SourceProductName=Computer Vision Toolbox  SourceProductBaseCode=VP
  Hough Transform : visiontransforms/Hough Transform  theta_res=pi/180  rho_res=1  out_theta_rho=on  outdtmode=single  roundingMode=Nearest  overflowMode=on  firstCoeffMode=Binary point scaling  firstCoeffWordLength=16  firstCoeffFracLength=14  firstCoeffSlope=2^-14  secondCoeffMode=Binary point scaling  secondCoeffWordLength=32  secondCoeffFracLength=16  secondCoeffSlope=2^-16  prodOutputMode=Binary point scaling  prodOutputWordLength=32  prodOutputFracLength=20  prodOutputSlope=2^-20  accumMode=Binary point scaling  accumWordLength=32  accumFracLength=20  accumSlope=2^-20  outputMode=Binary point scaling  outputWordLength=16  outputFracLength=0  outputSlope=2^0  memoryMode=Binary point scaling  memoryWordLength=32  memoryFracLength=16  memorySlope=2^-16
      settings: SourceProductName=Computer Vision Toolbox  SourceProductBaseCode=VP
  Overwrite Values : dspmtrx3/Overwrite Values  OverWriteDiag=Submatrix  valFrom2ndIP=Specify via dialog  ConstValue=0  RowSpan=All rows  RowStartMode=First  RowStartIndex=1  RowEndMode=Last  RowEndIndex=1  ColSpan=Range of columns  ColStartMode=First  ColStartIndex=1  ColEndMode=Index  ColEndIndex=20  DiagSpan=Range of elements  DiagStartMode=Index  DiagStartIndex=2  DiagEndMode=Index  DiagEndIndex=4
      settings: SourceProductName=DSP System Toolbox  SourceProductBaseCode=DS
  Overwrite Values1 : dspmtrx3/Overwrite Values  OverWriteDiag=Submatrix  valFrom2ndIP=Specify via dialog  ConstValue=0  RowSpan=All rows  RowStartMode=First  RowStartIndex=1  RowEndMode=Last  RowEndIndex=1  ColSpan=Range of columns  ColStartMode=Offset from last  ColStartIndex=20  ColEndMode=Last  ColEndIndex=15  DiagSpan=Range of elements  DiagStartMode=Index  DiagStartIndex=2  DiagEndMode=Index  DiagEndIndex=4
      settings: SourceProductName=DSP System Toolbox  SourceProductBaseCode=DS
  Peak detection : Subsystem
  Selector1 : Selector  NumberOfDimensions=2  InputPortWidth=3  IndexOptions=Index vector (dialog),Select all  Indices=[1],[2 1]  OutputSizes=1,1
  Selector2 : Selector  NumberOfDimensions=2  InputPortWidth=3  IndexOptions=Index vector (dialog),Select all  Indices=[2],[2 1]  OutputSizes=1,1
  Out1 : Outport
  wires:
  Overwrite Values/1 -> Overwrite Values1/1
  Hough Transform/1 -> Overwrite Values/1
  Hough Transform/2 -> Peak detection/2(Theta_list)
  Hough Transform/3 -> Peak detection/3(Rho_list)
  Peak detection/1(Line) -> Selector1/1, Selector2/1
  In1/1 -> Hough Transform/1
  ref_I/1 -> Hough Lines/3
  Hough Lines/1 -> Out1/1
  Overwrite Values1/1 -> Peak detection/1(Hough)
  Selector2/1 -> Hough Lines/1
  Selector1/1 -> Hough Lines/2

== system model/Vision-based Lane Detection Subsystem/Subsystem ==
  In1 : Inport
  Assignment : Assignment  NumberOfDimensions=2  DiagnosticForDimensions=Warning  IndexOptions=Index vector (dialog),Index vector (dialog)  Indices=1,3  OutputSizes=1,1
  Assignment1 : Assignment  NumberOfDimensions=2  DiagnosticForDimensions=Warning  IndexOptions=Index vector (dialog),Index vector (dialog)  Indices=2,3  OutputSizes=1,1
  Assignment2 : Assignment  NumberOfDimensions=2  DiagnosticForDimensions=Warning  IndexOptions=Index vector (dialog),Index vector (dialog)  Indices=1,4  OutputSizes=1,1
  Assignment3 : Assignment  NumberOfDimensions=2  DiagnosticForDimensions=Warning  IndexOptions=Index vector (dialog),Index vector (dialog)  Indices=2,4  OutputSizes=1,1
  Assignment4 : Assignment  NumberOfDimensions=2  DiagnosticForDimensions=Warning  IndexOptions=Index vector (dialog),Index vector (dialog)  Indices=1,1  OutputSizes=1,1
  Assignment5 : Assignment  NumberOfDimensions=2  DiagnosticForDimensions=Warning  IndexOptions=Index vector (dialog),Index vector (dialog)  Indices=2,1  OutputSizes=1,1
  Assignment6 : Assignment  NumberOfDimensions=2  DiagnosticForDimensions=Warning  IndexOptions=Index vector (dialog),Index vector (dialog)  Indices=1,2  OutputSizes=1,1
  Assignment7 : Assignment  NumberOfDimensions=2  DiagnosticForDimensions=Warning  IndexOptions=Index vector (dialog),Index vector (dialog)  Indices=2,2  OutputSizes=1,1
  Selector1 : Selector  NumberOfDimensions=2  InputPortWidth=3  IndexOptions=Index vector (dialog),Index vector (dialog)  Indices=2,3  OutputSizes=1,1
  Selector2 : Selector  NumberOfDimensions=2  InputPortWidth=3  IndexOptions=Index vector (dialog),Index vector (dialog)  Indices=2,4  OutputSizes=1,1
  Selector3 : Selector  NumberOfDimensions=2  InputPortWidth=3  IndexOptions=Index vector (dialog),Index vector (dialog)  Indices=1,4  OutputSizes=1,1
  Selector4 : Selector  NumberOfDimensions=2  InputPortWidth=3  IndexOptions=Index vector (dialog),Index vector (dialog)  Indices=2,1  OutputSizes=1,1
  Selector5 : Selector  NumberOfDimensions=2  InputPortWidth=3  IndexOptions=Index vector (dialog),Index vector (dialog)  Indices=1,3  OutputSizes=1,1
  Selector6 : Selector  NumberOfDimensions=2  InputPortWidth=3  IndexOptions=Index vector (dialog),Index vector (dialog)  Indices=1,1  OutputSizes=1,1
  Selector7 : Selector  NumberOfDimensions=2  InputPortWidth=3  IndexOptions=Index vector (dialog),Index vector (dialog)  Indices=2,2  OutputSizes=1,1
  Selector8 : Selector  NumberOfDimensions=2  InputPortWidth=3  IndexOptions=Index vector (dialog),Index vector (dialog)  Indices=1,2  OutputSizes=1,1
  Switch{1..8} (8 alike) : Switch  Criteria=u2 > Threshold  Threshold=100
  Out1 : Outport
  wires:
  Switch5/1 -> Assignment4/2
  Assignment7/1 -> Out1/1
  Switch8/1 -> Assignment7/2
  Assignment6/1 -> Assignment7/1
  Switch7/1 -> Assignment6/2
  Assignment5/1 -> Assignment6/1
  Selector8/1 -> Switch7/3, Switch8/1
  Selector7/1 -> Switch7/1, Switch8/3
  Switch6/1 -> Assignment5/2
  Assignment4/1 -> Assignment5/1
  Assignment3/1 -> Assignment4/1
  Selector6/1 -> Switch5/3, Switch6/1
  Selector4/1 -> Switch5/1, Switch6/3
  Switch4/1 -> Assignment3/2
  Assignment2/1 -> Assignment3/1
  Switch3/1 -> Assignment2/2
  Selector3/1 -> Switch3/3, Switch4/1
  Selector2/1 -> Switch3/1, Switch4/3
  Assignment1/1 -> Assignment2/1
  Switch1/1 -> Assignment1/2
  Assignment/1 -> Assignment1/1
  In1/1 -> Selector5/1, Assignment/1, Selector1/1, Selector2/1, Selector3/1, Selector4/1, Selector6/1, Selector7/1, Selector8/1
  Switch2/1 -> Assignment/2
  Selector1/1 -> Switch2/1, Switch1/3
  Selector5/1 -> Switch2/2, Switch2/3, Switch1/1, Switch1/2, Switch3/2, Switch4/2, Switch5/2, Switch6/2, Switch7/2, Switch8/2

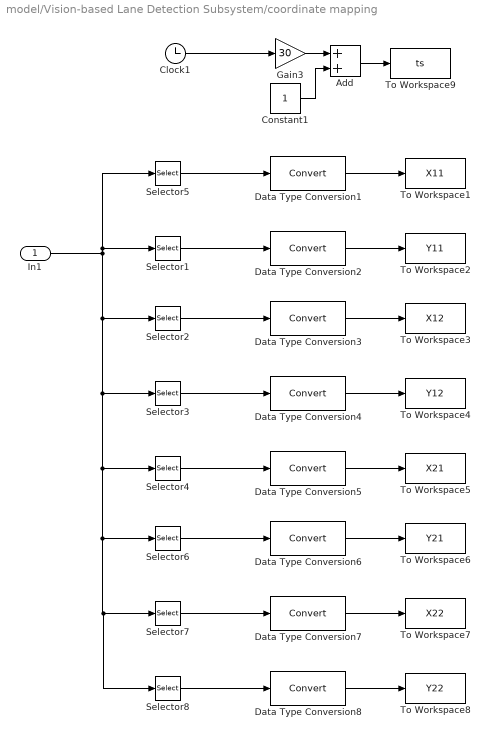
== system model/Vision-based Lane Detection Subsystem/coordinate mapping ==
  In1 : Inport
  Add : Sum
  Clock1 : Clock
  Constant1 : Constant
  Data Type Conversion{1..8} (8 alike) : DataTypeConversion
  Gain3 : Gain  Gain=30
  Selector1 : Selector  NumberOfDimensions=2  InputPortWidth=3  IndexOptions=Index vector (dialog),Index vector (dialog)  Indices=1,2  OutputSizes=1,1
  Selector2 : Selector  NumberOfDimensions=2  InputPortWidth=3  IndexOptions=Index vector (dialog),Index vector (dialog)  Indices=1,3  OutputSizes=1,1
  Selector3 : Selector  NumberOfDimensions=2  InputPortWidth=3  IndexOptions=Index vector (dialog),Index vector (dialog)  Indices=1,4  OutputSizes=1,1
  Selector4 : Selector  NumberOfDimensions=2  InputPortWidth=3  IndexOptions=Index vector (dialog),Index vector (dialog)  Indices=2,1  OutputSizes=1,1
  Selector5 : Selector  NumberOfDimensions=2  InputPortWidth=3  IndexOptions=Index vector (dialog),Index vector (dialog)  Indices=1,1  OutputSizes=1,1
  Selector6 : Selector  NumberOfDimensions=2  InputPortWidth=3  IndexOptions=Index vector (dialog),Index vector (dialog)  Indices=2,2  OutputSizes=1,1
  Selector7 : Selector  NumberOfDimensions=2  InputPortWidth=3  IndexOptions=Index vector (dialog),Index vector (dialog)  Indices=2,3  OutputSizes=1,1
  Selector8 : Selector  NumberOfDimensions=2  InputPortWidth=3  IndexOptions=Index vector (dialog),Index vector (dialog)  Indices=2,4  OutputSizes=1,1
  To Workspace1 : ToWorkspace  VariableName=X11  SampleTime=-1
      settings: Save2DSignal=2-D array (concatenate along first dimension)
  To Workspace2 : ToWorkspace  VariableName=Y11  SampleTime=-1
      settings: Save2DSignal=2-D array (concatenate along first dimension)
  To Workspace3 : ToWorkspace  VariableName=X12  SampleTime=-1
      settings: Save2DSignal=2-D array (concatenate along first dimension)
  To Workspace4 : ToWorkspace  VariableName=Y12  SampleTime=-1
      settings: Save2DSignal=2-D array (concatenate along first dimension)
  To Workspace5 : ToWorkspace  VariableName=X21  SampleTime=-1
      settings: Save2DSignal=2-D array (concatenate along first dimension)
  To Workspace6 : ToWorkspace  VariableName=Y21  SampleTime=-1
      settings: Save2DSignal=2-D array (concatenate along first dimension)
  To Workspace7 : ToWorkspace  VariableName=X22  SampleTime=-1
      settings: Save2DSignal=2-D array (concatenate along first dimension)
  To Workspace8 : ToWorkspace  VariableName=Y22  SampleTime=-1
      settings: Save2DSignal=2-D array (concatenate along first dimension)
  To Workspace9 : ToWorkspace  VariableName=ts  SampleTime=-1
  wires:
  Data Type Conversion2/1 -> To Workspace2/1
  Data Type Conversion1/1 -> To Workspace1/1
  In1/1 -> Selector1/1, Selector5/1, Selector8/1, Selector7/1, Selector6/1, Selector4/1, Selector3/1, Selector2/1
  Selector5/1 -> Data Type Conversion1/1
  Selector1/1 -> Data Type Conversion2/1
  Data Type Conversion3/1 -> To Workspace3/1
  Data Type Conversion4/1 -> To Workspace4/1
  Selector3/1 -> Data Type Conversion4/1
  Selector2/1 -> Data Type Conversion3/1
  Data Type Conversion5/1 -> To Workspace5/1
  Selector4/1 -> Data Type Conversion5/1
  Data Type Conversion6/1 -> To Workspace6/1
  Data Type Conversion7/1 -> To Workspace7/1
  Data Type Conversion8/1 -> To Workspace8/1
  Selector6/1 -> Data Type Conversion6/1
  Selector7/1 -> Data Type Conversion7/1
  Selector8/1 -> Data Type Conversion8/1
  Constant1/1 -> Add/2
  Add/1 -> To Workspace9/1
  Clock1/1 -> Gain3/1
  Gain3/1 -> Add/1

== system model/Vision-based Lane Detection Subsystem/lateral offset ==
  right : Inport
  left : Inport  Port=2
  Abs : Abs
  Abs1 : Abs
  Add : Sum  Inputs=+-
  Add2 : Sum  Inputs=-+
  Add3 : Sum  Inputs=+-
  Divide : Product  Inputs=*/
  Gain1 : Gain  Gain=0.8
  MinMax : MinMax  Inputs=2
  Saturation : Saturate  UpperLimit=176  LowerLimit=0
  half width : Constant  Value=160
  lateral offset : Outport
  wires:
  half width/1 -> Add2/1, Gain1/1, Add/1
  right/1 -> Add2/2
  MinMax/1 -> Saturation/1
  Gain1/1 -> Divide/2, Add3/2
  Saturation/1 -> Add3/1
  Add3/1 -> Divide/1
  Divide/1 -> lateral offset/1
  left/1 -> Add/2
  Add2/1 -> Abs/1
  Add/1 -> Abs1/1
  Abs/1 -> MinMax/1
  Abs1/1 -> MinMax/2

== system model/Vision-based Lane Detection Subsystem/offset (+88) ==
  In1 : Inport
  Assignment : Assignment  NumberOfDimensions=2  DiagnosticForDimensions=Warning  IndexOptions=Index vector (dialog),Index vector (dialog)  Indices=1,1  OutputSizes=1,1
  Assignment1 : Assignment  NumberOfDimensions=2  DiagnosticForDimensions=Warning  IndexOptions=Index vector (dialog),Index vector (dialog)  Indices=3,1  OutputSizes=1,1
  Assignment2 : Assignment  NumberOfDimensions=2  DiagnosticForDimensions=Warning  IndexOptions=Index vector (dialog),Index vector (dialog)  Indices=3,2  OutputSizes=1,1
  Assignment3 : Assignment  NumberOfDimensions=2  DiagnosticForDimensions=Warning  IndexOptions=Index vector (dialog),Index vector (dialog)  Indices=1,2  OutputSizes=1,1
  Assignment4 : Assignment  NumberOfDimensions=2  DiagnosticForDimensions=Warning  IndexOptions=Index vector (dialog),Index vector (dialog)  Indices=2,2  OutputSizes=1,1
  Assignment5 : Assignment  NumberOfDimensions=2  DiagnosticForDimensions=Warning  IndexOptions=Index vector (dialog),Index vector (dialog)  Indices=2,1  OutputSizes=1,1
  Bias{,1..3} (4 alike) : Bias  Bias=u
  Selector1 : Selector  NumberOfDimensions=2  InputPortWidth=3  IndexOptions=Index vector (dialog),Index vector (dialog)  Indices=4,2  OutputSizes=1,1
  Selector2 : Selector  NumberOfDimensions=2  InputPortWidth=3  IndexOptions=Index vector (dialog),Index vector (dialog)  Indices=4,1  OutputSizes=1,1
  Selector3 : Selector  NumberOfDimensions=2  InputPortWidth=3  IndexOptions=Index vector (dialog),Index vector (dialog)  Indices=2,2  OutputSizes=1,1
  Selector4 : Selector  NumberOfDimensions=2  InputPortWidth=3  IndexOptions=Index vector (dialog),Index vector (dialog)  Indices=2,1  OutputSizes=1,1
  Selector5 : Selector  NumberOfDimensions=2  InputPortWidth=3  IndexOptions=Index vector (dialog),Index vector (dialog)  Indices=1,1  OutputSizes=1,1
  Selector6 : Selector  NumberOfDimensions=2  InputPortWidth=3  IndexOptions=Index vector (dialog),Index vector (dialog)  Indices=3,1  OutputSizes=1,1
  Selector7 : Selector  NumberOfDimensions=2  InputPortWidth=3  IndexOptions=Index vector (dialog),Index vector (dialog)  Indices=3,2  OutputSizes=1,1
  Selector8 : Selector  NumberOfDimensions=2  InputPortWidth=3  IndexOptions=Index vector (dialog),Index vector (dialog)  Indices=1,2  OutputSizes=1,1
  Out1 : Outport
  left : Outport  Port=2
  right : Outport  Port=3
  wires:
  Selector5/1 -> Bias/1
  Bias/1 -> Assignment/2
  Assignment/1 -> Selector6/1, Assignment1/1
  Selector6/1 -> Bias1/1
  Bias1/1 -> Assignment1/2
  Assignment1/1 -> Selector7/1, Assignment2/1
  Selector7/1 -> Bias2/1
  Bias2/1 -> Assignment2/2
  Assignment2/1 -> Selector8/1, Assignment3/1
  Selector8/1 -> Bias3/1
  Bias3/1 -> Assignment3/2
  Selector2/1 -> right/1
  Selector1/1 -> left/1
  Assignment3/1 -> Selector3/1, Assignment4/1
  Assignment4/1 -> Selector4/1, Assignment5/1
  In1/1 -> Assignment/1, Selector5/1
  Assignment5/1 -> Selector2/1, Selector1/1, Out1/1
  Selector4/1 -> Assignment5/2
  Selector3/1 -> Assignment4/2

== system model/Model-based Vehicle Model Subsystem/Brake // Traction Torques1/BRAKE ==
  Demux : Demux  Tag=STV Demux  Outputs=1
  FromWs : FromWorkspace  Tag=STV FromWs  VariableName=tuvar  SampleTime=0
      SigBuilderData=|
      | common.afterFinalStr = 'Extrapolate'
      | common.sampleTime = 0
      | dataSet.timeRange = [0 10]
      | dataSet.name = 'Group 1'
      | sbobj.Groups.Name = 'Group 1'
      | sbobj.Groups.Signals.Name = 'Signal 1'
      | sbobj.Groups.Signals.XData = [0 2 2.1 10]
      | sbobj.Groups.Signals.YData = [0 0 1 1]
  Signal 1 : Outport  Tag=STV Outport
  wires:
  FromWs/1 -> Demux/1
  Demux/1 -> Signal 1/1

== system model/Model-based Vehicle Model Subsystem/Brake // Traction Torques1/THROTTLE1 ==
  Demux : Demux  Tag=STV Demux  Outputs=1
  FromWs : FromWorkspace  Tag=STV FromWs  VariableName=tuvar  SampleTime=0
      SigBuilderData=|
      | common.afterFinalStr = 'Extrapolate'
      | common.sampleTime = 0
      | dataSet.timeRange = [0 10]
      | dataSet.name = 'Group 1'
      | sbobj.Groups.Name = 'Group 1'
      | sbobj.Groups.Signals.Name = 'Signal 1'
      | sbobj.Groups.Signals.XData = [0 1 1.1 1.9 2 10]
      | sbobj.Groups.Signals.YData = [0 0 1 1 1 1]
  Signal 1 : Outport  Tag=STV Outport
  wires:
  FromWs/1 -> Demux/1
  Demux/1 -> Signal 1/1

== system model/Model-based Vehicle Model Subsystem/Handling Model /Lateral  ==
  Steer : Inport
  Fxfl : Inport  Port=2
  Fyfl : Inport  Port=3
  Fxfr : Inport  Port=4
  Fyfr : Inport  Port=5
  Fyrl : Inport  Port=6
  Fyrr : Inport  Port=7
  Add : Sum
  Add1 : Sum  Inputs=+++
  Add2 : Sum
  Add3 : Sum
  Gain : Gain  Gain=1/m
  Product : Product  RndMeth=Zero
  Product1 : Product  RndMeth=Zero
  Trigonometric Function : Trigonometry
  Trigonometric Function1 : Trigonometry  Operator=cos
  ay : Outport
  wires:
  Fyrl/1 -> Add/1
  Fyrr/1 -> Add/2
  Steer/1 -> Trigonometric Function/1, Trigonometric Function1/1
  Add/1 -> Add1/3
  Fyfl/1 -> Add3/1
  Fyfr/1 -> Add3/2
  Trigonometric Function1/1 -> Product/1
  Add3/1 -> Product/2
  Product/1 -> Add1/2
  Fxfr/1 -> Add2/2
  Fxfl/1 -> Add2/1
  Add2/1 -> Product1/1
  Trigonometric Function/1 -> Product1/2
  Product1/1 -> Add1/1
  Add1/1 -> Gain/1
  Gain/1 -> ay/1

== system model/Model-based Vehicle Model Subsystem/Handling Model /Longitudinal  ==
  Steer : Inport
  Fxfl : Inport  Port=2
  Fyfl : Inport  Port=3
  Fxfr : Inport  Port=4
  Fyfr : Inport  Port=5
  Fxrl : Inport  Port=6
  Fxrr : Inport  Port=7
  Add : Sum  Inputs=++-
  Add1 : Sum
  Add2 : Sum
  Add3 : Sum
  Gain : Gain  Gain=1/m
  Product : Product  RndMeth=Zero
  Product1 : Product  RndMeth=Zero
  Trigonometric Function : Trigonometry
  Trigonometric Function1 : Trigonometry  Operator=cos
  ax : Outport
  wires:
  Fxrr/1 -> Add1/1
  Add1/1 -> Add/1
  Steer/1 -> Trigonometric Function/1, Trigonometric Function1/1
  Trigonometric Function/1 -> Product/1
  Fxrl/1 -> Add1/2
  Fyfl/1 -> Add2/1
  Fyfr/1 -> Add2/2
  Add2/1 -> Product/2
  Product/1 -> Add/3
  Fxfl/1 -> Add3/1
  Fxfr/1 -> Add3/2
  Trigonometric Function1/1 -> Product1/1
  Add3/1 -> Product1/2
  Product1/1 -> Add/2
  Add/1 -> Gain/1
  Gain/1 -> ax/1

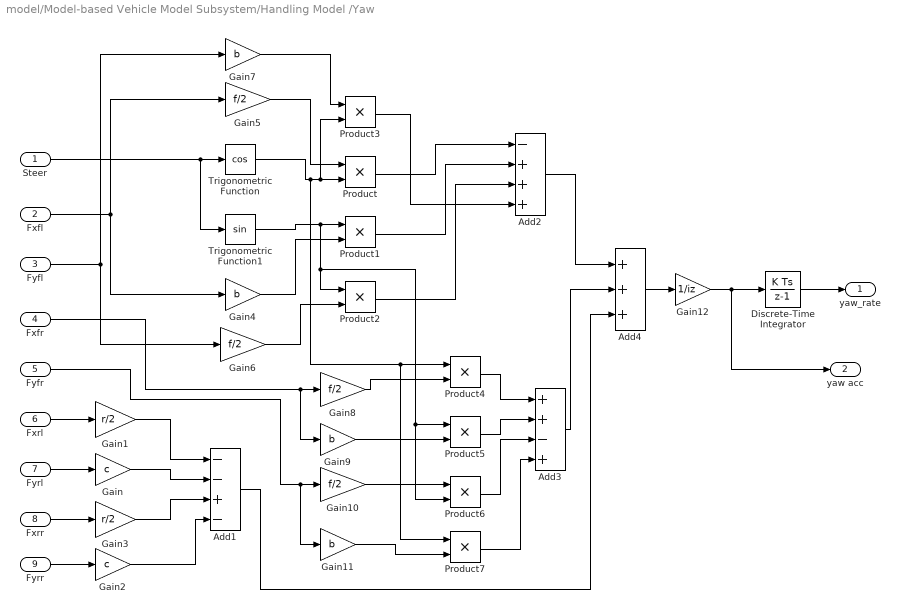
== system model/Model-based Vehicle Model Subsystem/Handling Model /Yaw   ==
  Steer : Inport
  Fxfl : Inport  Port=2
  Fyfl : Inport  Port=3
  Fxfr : Inport  Port=4
  Fyfr : Inport  Port=5
  Fxrl : Inport  Port=6
  Fyrl : Inport  Port=7
  Fxrr : Inport  Port=8
  Fyrr : Inport  Port=9
  Add1 : Sum  Inputs=--+-
  Add2 : Sum  Inputs=-+++
  Add3 : Sum  Inputs=++-+
  Add4 : Sum  Inputs=+++
  Discrete-Time Integrator : DiscreteIntegrator  SampleTime=-1  ICPrevOutput=DiscIntNeverNeededParam  ICPrevScaledInput=DiscIntNeverNeededParam
  Gain : Gain  Gain=c
  Gain1 : Gain  Gain=r/2
  Gain{5..6,8,10} (4 alike) : Gain  Gain=f/2
  Gain{4,7,9,11} (4 alike) : Gain  Gain=b
  Gain12 : Gain  Gain=1/iz
  Gain2 : Gain  Gain=c
  Gain3 : Gain  Gain=r/2
  Product{,1..7} (8 alike) : Product  RndMeth=Zero
  Trigonometric Function : Trigonometry  Operator=cos
  Trigonometric Function1 : Trigonometry
  yaw_rate : Outport
  yaw acc : Outport  Port=2
  wires:
  Fyrl/1 -> Gain/1
  Fxrl/1 -> Gain1/1
  Fyrr/1 -> Gain2/1
  Fxrr/1 -> Gain3/1
  Gain1/1 -> Add1/1
  Gain/1 -> Add1/2
  Gain3/1 -> Add1/3
  Gain2/1 -> Add1/4
  Steer/1 -> Trigonometric Function/1, Trigonometric Function1/1
  Trigonometric Function/1 -> Product/2, Product3/2, Product4/1, Product7/1
  Fxfl/1 -> Gain5/1, Gain4/1
  Gain5/1 -> Product/1
  Product/1 -> Add2/1
  Trigonometric Function1/1 -> Product1/1, Product2/1, Product5/1, Product6/2
  Gain4/1 -> Product1/2
  Product1/1 -> Add2/2
  Gain6/1 -> Product2/2
  Fyfl/1 -> Gain6/1, Gain7/1
  Product2/1 -> Add2/3
  Gain7/1 -> Product3/1
  Product3/1 -> Add2/4
  Fxfr/1 -> Gain8/1, Gain9/1
  Gain8/1 -> Product4/2
  Product4/1 -> Add3/1
  Gain9/1 -> Product5/2
  Product5/1 -> Add3/2
  Gain10/1 -> Product6/1
  Fyfr/1 -> Gain10/1, Gain11/1
  Product6/1 -> Add3/3
  Gain11/1 -> Product7/2
  Product7/1 -> Add3/4
  Add2/1 -> Add4/1
  Add3/1 -> Add4/2
  Add1/1 -> Add4/3
  Discrete-Time Integrator/1 -> yaw_rate/1
  Add4/1 -> Gain12/1
  Gain12/1 -> yaw acc/1, Discrete-Time Integrator/1
